simulink model "Demo"  (R2023a)
settings: Solver=VariableStepAuto  StartTime=0.0  StopTime=10.0  RelTol=1e-3
settings Model: Creator=nikit  LastModifiedBy=nikit

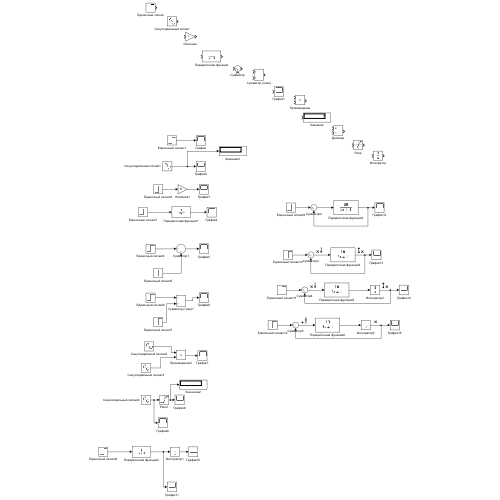
[thumbnail: Simulink's stored preview of the top-level diagram]
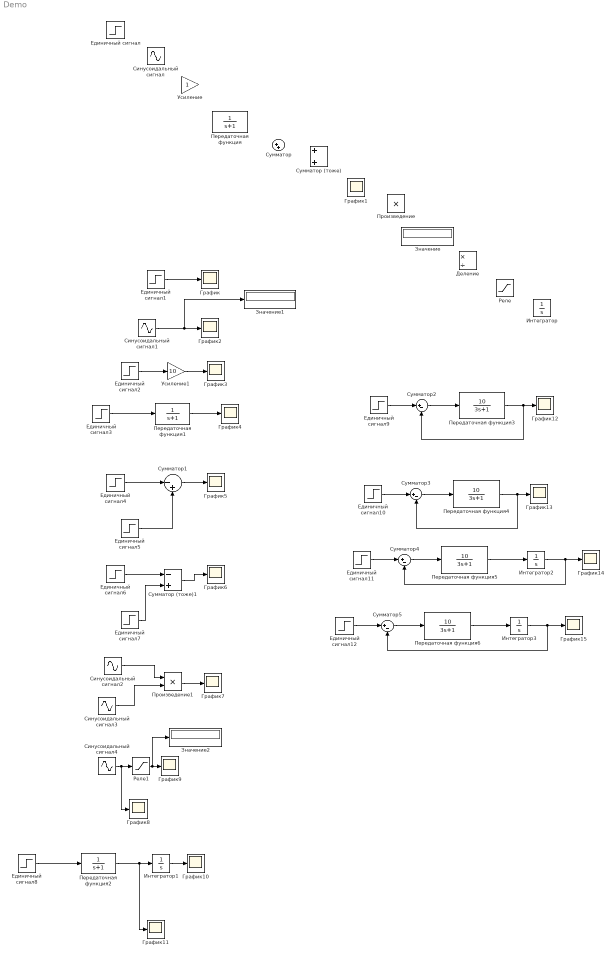
== system Demo ==
  График{,1..15} (16 alike) : Scope
  Деление : Product  Inputs=*/
  Единичный сигнал : Step  SampleTime=0
  Единичный сигнал1 : Step  Time=4  After=3  SampleTime=0
  Единичный сигнал{2..3,8..12} (7 alike) : Step  Time=0  SampleTime=0
  Единичный сигнал4 : Step  Time=0  After=3  SampleTime=0
  Единичный сигнал5 : Step  Time=2  After=4  SampleTime=0
  Единичный сигнал6 : Step  Time=0  After=3  SampleTime=0
  Единичный сигнал7 : Step  Time=2  After=4  SampleTime=0
  Значение : Display
  Значение1 : Display
  Значение2 : Display
  Интегратор{,1..3} (4 alike) : Integrator
  Передаточная функция : TransferFcn  Denominator=[1 1]
  Передаточная функция1 : TransferFcn  Denominator=[1 1]
  Передаточная функция2 : TransferFcn  Denominator=[1 1]
  Передаточная функция{3..6} (4 alike) : TransferFcn  Numerator=[10]  Denominator=[3 1]
  Произведение : Product
  Произведение1 : Product
  Реле : Saturate
  Реле1 : Saturate
  Синусоидальный сигнал : Sin  SampleTime=0
  Синусоидальный сигнал1 : Sin  Frequency=2  SampleTime=0
  Синусоидальный сигнал2 : Sin  Amplitude=3  Bias=10  Frequency=0.5  Phase=2  SampleTime=0
  Синусоидальный сигнал3 : Sin  Frequency=2  SampleTime=0
  Синусоидальный сигнал4 : Sin  Frequency=2  SampleTime=0
  Сумматор : Sum  Inputs=|++
  Сумматор (тоже) : Sum
  Сумматор (тоже)1 : Sum  Inputs=-+
  Сумматор1 : Sum  Inputs=|-+
  Сумматор{2..5} (4 alike) : Sum  Inputs=|+-
  Усиление : Gain
  Усиление1 : Gain  Gain=10
  wires:
  Единичный сигнал1/1 -> График/1
  Единичный сигнал2/1 -> Усиление1/1
  Усиление1/1 -> График3/1
  Единичный сигнал3/1 -> Передаточная функция1/1
  Передаточная функция1/1 -> График4/1
  Единичный сигнал4/1 -> Сумматор1/1
  Единичный сигнал5/1 -> Сумматор1/2
  Сумматор1/1 -> График5/1
  Сумматор (тоже)1/1 -> График6/1
  Единичный сигнал7/1 -> Сумматор (тоже)1/2
  Единичный сигнал6/1 -> Сумматор (тоже)1/1
  Синусоидальный сигнал2/1 -> Произведение1/1
  Синусоидальный сигнал3/1 -> Произведение1/2
  Произведение1/1 -> График7/1
  Синусоидальный сигнал1/1 -> Значение1/1, График2/1
  Синусоидальный сигнал4/1 -> График8/1, Реле1/1
  Реле1/1 -> Значение2/1, График9/1
  Единичный сигнал8/1 -> Передаточная функция2/1
  Передаточная функция2/1 -> График11/1, Интегратор1/1
  Интегратор1/1 -> График10/1
  Передаточная функция3/1 -> График12/1, Сумматор2/2
  Единичный сигнал9/1 -> Сумматор2/1
  Сумматор2/1 -> Передаточная функция3/1
  Передаточная функция4/1 -> График13/1, Сумматор3/2
  Единичный сигнал10/1 -> Сумматор3/1
  Сумматор3/1 -> Передаточная функция4/1
  Передаточная функция5/1 -> Интегратор2/1
  Единичный сигнал11/1 -> Сумматор4/1
  Сумматор4/1 -> Передаточная функция5/1
  Интегратор2/1 -> Сумматор4/2, График14/1
  Интегратор3/1 -> Сумматор5/2, График15/1
  Сумматор5/1 -> Передаточная функция6/1
  Передаточная функция6/1 -> Интегратор3/1
  Единичный сигнал12/1 -> Сумматор5/1
